simulink model "TAYLOR_TYPE_ZNNU"  (R2024a)
settings: Solver=ode4  StartTime=0.0  StopTime=10.0  FixedStep=0.01  RelTol=1e-3
values from neighbouring files (symbols this model uses):
  h = tau*gamma    (= 0.4)    [setup.m]
  u0 = ones(3, 1)    [setup.m]
  u1 = ones(3, 1)    [setup.m]
  W0 = ones(3)    [setup.m]
  W1 = ones(3)    [setup.m]
  y0 = ones(3, 1)    [setup.m]
  y1 = ones(3, 1)    [setup.m]
  y2 = ones(3, 1)    [setup.m]
settings Model: Creator=uli_2  LastModifiedBy=uli_2
settings DebuggingCC: UnconnectedInputMsg=warning  UnconnectedOutputMsg=warning  UnconnectedLineMsg=warning
settings ModelReferenceCC: EnableRefExpFcnMdlSchedulingChecks=on
settings RTWCC: GPUComputeCapability=3.5  DLArmComputeVersion=19.05

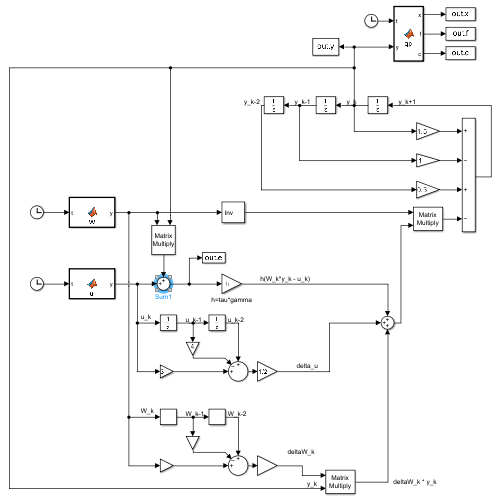
[thumbnail: Simulink's stored preview of the top-level diagram]
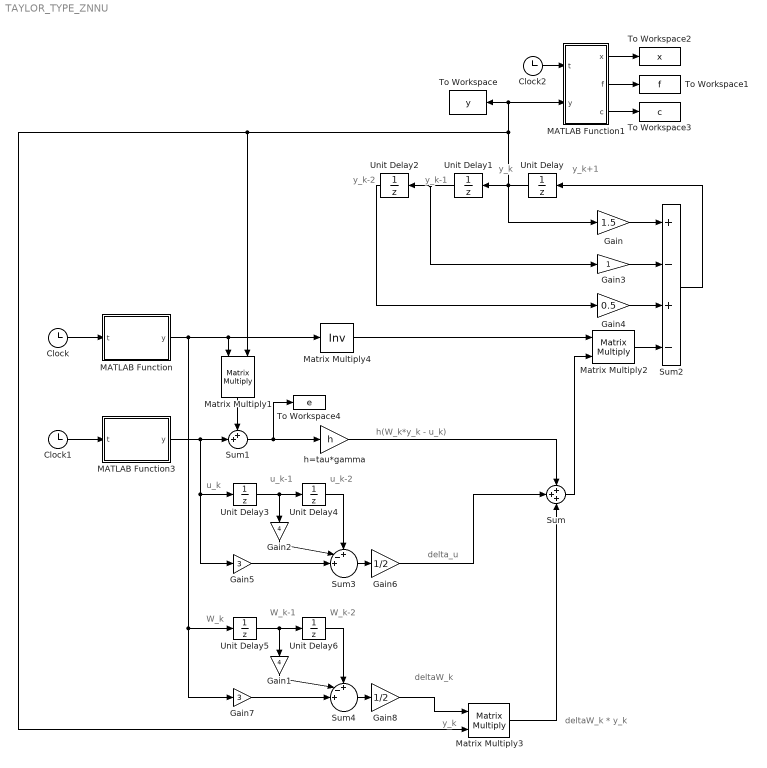
== system TAYLOR_TYPE_ZNNU ==
  note: y_k
  note: delta_u
  note: u_k-2
  note: u_k-1
  note: u_k
  note: deltaW_k
  note: y_k
  note: h(W_k*y_k - u_k)
  note: y_k-2
  note: deltaW_k * y_k
  note: y_k+1
  note: y_k-1
  note: W_k-2
  note: W_k-1
  note: W_k
  Clock : Clock
  Clock1 : Clock
  Clock2 : Clock
  Gain : Gain  Gain=1.5
  Gain1 : Gain  Gain=4
  Gain2 : Gain  Gain=4
  Gain3 : Gain
  Gain4 : Gain  Gain=0.5
  Gain5 : Gain  Gain=3
  Gain6 : Gain  Gain=1/2
  Gain7 : Gain  Gain=3
  Gain8 : Gain  Gain=1/2
  MATLAB Function : MATLAB Function  TreatAsAtomicUnit=on
  MATLAB Function1 : MATLAB Function  TreatAsAtomicUnit=on
  MATLAB Function3 : MATLAB Function  TreatAsAtomicUnit=on
  Matrix Multiply1 : Product  Multiplication=Matrix(*)
  Matrix Multiply2 : Product  Multiplication=Matrix(*)
  Matrix Multiply3 : Product  Multiplication=Matrix(*)
  Matrix Multiply4 : Product  Inputs=/  Multiplication=Matrix(*)
  Sum : Sum  Inputs=+++
  Sum1 : Sum  Inputs=++|
  Sum2 : Sum  Inputs=+-+-
  Sum3 : Sum  Inputs=+-+||
  Sum4 : Sum  Inputs=+-+||
  To Workspace : ToWorkspace  VariableName=y  SaveFormat=Timeseries  SampleTime=-1
  To Workspace1 : ToWorkspace  VariableName=f  SaveFormat=Timeseries  SampleTime=-1
  To Workspace2 : ToWorkspace  VariableName=x  SaveFormat=Timeseries  SampleTime=-1
  To Workspace3 : ToWorkspace  VariableName=c  SaveFormat=Timeseries  SampleTime=-1
  To Workspace4 : ToWorkspace  VariableName=e  SaveFormat=Timeseries  SampleTime=-1
  Unit Delay : UnitDelay  InitialCondition=y2  SampleTime=-1  HasFrameUpgradeWarning=on
  Unit Delay1 : UnitDelay  InitialCondition=y1  SampleTime=-1  HasFrameUpgradeWarning=on
  Unit Delay2 : UnitDelay  InitialCondition=y0  SampleTime=-1  HasFrameUpgradeWarning=on
  Unit Delay3 : UnitDelay  InitialCondition=u1  SampleTime=-1  HasFrameUpgradeWarning=on
  Unit Delay4 : UnitDelay  InitialCondition=u0  SampleTime=-1  HasFrameUpgradeWarning=on
  Unit Delay5 : UnitDelay  InitialCondition=W1  SampleTime=-1  HasFrameUpgradeWarning=on
  Unit Delay6 : UnitDelay  InitialCondition=W0  SampleTime=-1  HasFrameUpgradeWarning=on
  h=tau*gamma : Gain  Gain=h
  wires:
  Matrix Multiply4/1 -> Matrix Multiply2/1
  Gain4/1 -> Sum2/3
  Sum2/1 -> Unit Delay/1
  MATLAB Function1/2(f) -> To Workspace1/1
  Unit Delay2/1 -> Gain4/1
  MATLAB Function1/1(x) -> To Workspace2/1
  Sum/1 -> Matrix Multiply2/2
  Matrix Multiply2/1 -> Sum2/4
  Gain/1 -> Sum2/1
  Sum1/1 -> To Workspace4/1, h=tau*gamma/1
  Clock/1 -> MATLAB Function/1(t)
  Unit Delay/1 -> Gain/1, MATLAB Function1/2(y), To Workspace/1, Matrix Multiply1/2, Matrix Multiply3/2, Unit Delay1/1
  Matrix Multiply3/1 -> Sum/3
  Unit Delay1/1 -> Gain3/1, Unit Delay2/1
  Clock1/1 -> MATLAB Function3/1(t)
  h=tau*gamma/1 -> Sum/1
  MATLAB Function1/3(c) -> To Workspace3/1
  Clock2/1 -> MATLAB Function1/1(t)
  Gain3/1 -> Sum2/2
  Matrix Multiply1/1 -> Sum1/1
  Unit Delay3/1 -> Unit Delay4/1, Gain2/1
  Unit Delay4/1 -> Sum3/1
  Gain2/1 -> Sum3/2
  Gain5/1 -> Sum3/3
  MATLAB Function3/1(y) -> Sum1/2, Unit Delay3/1, Gain5/1
  Sum3/1 -> Gain6/1
  Gain6/1 -> Sum/2
  Sum4/1 -> Gain8/1
  MATLAB Function/1(y) -> Matrix Multiply4/1, Matrix Multiply1/1, Unit Delay5/1, Gain7/1
  Gain7/1 -> Sum4/3
  Gain1/1 -> Sum4/2
  Unit Delay6/1 -> Sum4/1
  Unit Delay5/1 -> Gain1/1, Unit Delay6/1
  Gain8/1 -> Matrix Multiply3/1

== matlab function TAYLOR_TYPE_ZNNU/MATLAB Function1 ==
  data: t input; y input; x output; f output; c output
function [x,f,c] = qp(t, y)
    n = 2;
    x = y(1:n); lambda = y(n+1:end);
    P = [sin(t)/4 + 1, cos(t)/2; cos(t)/2, cos(t)/4 + 1];
    A = [sin(4*t), cos(4*t)];
    q = [sin(3*t); cos(3*t)];
    b = cos(2*t);
    f = x' * P * x + q' * x;
    c = A * x - b;

== matlab function TAYLOR_TYPE_ZNNU/MATLAB Function ==
  data: t input; y output
function y = W(t)
    m = 1;
    P = [sin(t)/4 + 1, cos(t)/2; cos(t)/2, cos(t)/4 + 1];
    A = [sin(4*t), cos(4*t)];
    y = [P, A'; A, zeros(m)];

== matlab function TAYLOR_TYPE_ZNNU/MATLAB Function3 ==
  data: t input; y output
function y = u(t)
    q = [sin(3*t); cos(3*t)];
    b = cos(2*t);
    y = [q; -b];
